simulink model "stg3"  (Simulink 7.0)
settings: Solver=ode45  StartTime=0.0  StopTime=100  RelTol=1e-3
libraries: xbsIndex_r4 x243, xps_library x11, casper_library x4
(part 1 of 2)
settings Model: Creator=dave  LastModifiedBy=dave

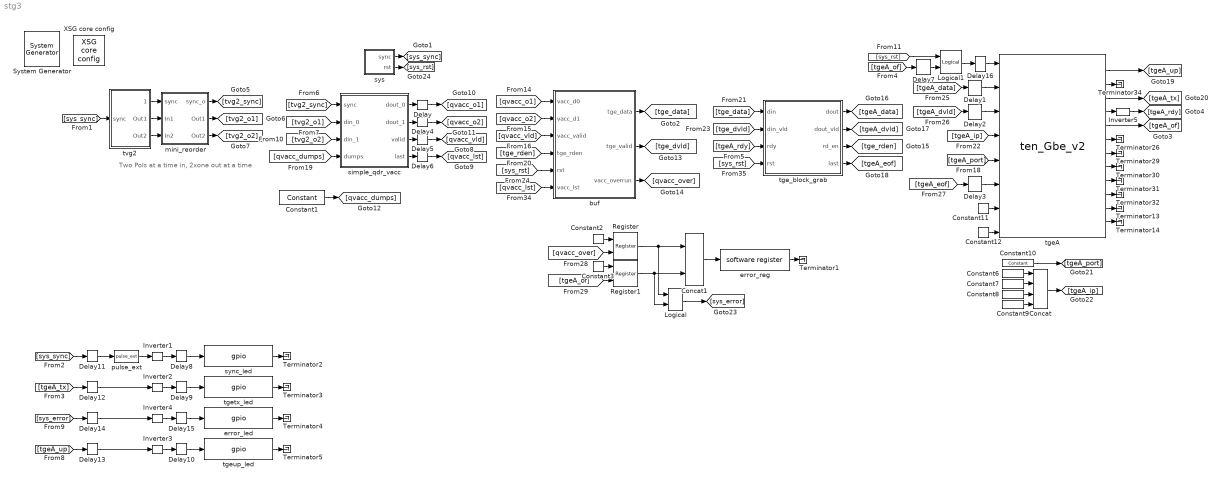
== system stg3 ==
  note: Two Pols at a time in,
      | 2xone out at a time
  " System Generator" : xbsIndex_r4/ System Generator  Tag=genX  SystemSampleTime=-1  xilinxfamily=virtex5  part=xc5vsx95t  speed=-1  package=ff1136  synthesis_tool=XST  clock_wrapper=Clock Enables  directory=./stg3/sysgen  testbench=off  simulink_period=1  sysclk_period=3.3333  dcm_input_clock_period=100  incr_netlist=off  trim_vbits=Everywhere in SubSystem  dbl_ovrd=According to Block Masks  core_generation=According to Block Masks  run_coregen=off  deprecated_control=off  eval_field=0  block_type=sysgen
      settings: block_version=10.1.3
  Concat : xbsIndex_r4/Concat  num_inputs=4  dbl_ovrd=off  block_type=concat
      settings: block_version=10.1.3
  Concat1 : xbsIndex_r4/Concat  num_inputs=2  dbl_ovrd=off  block_type=concat
      settings: block_version=10.1.3
  Constant1 : xbsIndex_r4/Constant  arith_type=Unsigned  const=(2^10)*(2^(10-1))*(2^9) - 2  n_bits=32  bin_pt=0  explicit_period=on  period=1  equ=P=C  opselect=C  inp2=PCIN>>17  opr=+  inp1=P  carry=CIN  dbl_ovrd=off  block_type=constant
  Constant10 : xbsIndex_r4/Constant  arith_type=Unsigned  const=10000  n_bits=16  bin_pt=0  explicit_period=off  period=1  equ=P=C  opselect=C  inp2=PCIN>>17  opr=+  inp1=P  carry=CIN  dbl_ovrd=off  block_type=constant
  Constant{2..3,11..12} (4 alike) : xbsIndex_r4/Constant  arith_type=Boolean  const=1  n_bits=16  bin_pt=14  explicit_period=off  period=1  equ=P=C  opselect=C  inp2=PCIN>>17  opr=+  inp1=P  carry=CIN  dbl_ovrd=off  block_type=constant
  Constant6 : xbsIndex_r4/Constant  arith_type=Unsigned  const=192  n_bits=8  bin_pt=0  explicit_period=off  period=1  equ=P=C  opselect=C  inp2=PCIN>>17  opr=+  inp1=P  carry=CIN  dbl_ovrd=off  block_type=constant
  Constant7 : xbsIndex_r4/Constant  arith_type=Unsigned  const=168  n_bits=8  bin_pt=0  explicit_period=off  period=1  equ=P=C  opselect=C  inp2=PCIN>>17  opr=+  inp1=P  carry=CIN  dbl_ovrd=off  block_type=constant
  Constant8 : xbsIndex_r4/Constant  arith_type=Unsigned  const=5  n_bits=8  bin_pt=0  explicit_period=off  period=1  equ=P=C  opselect=C  inp2=PCIN>>17  opr=+  inp1=P  carry=CIN  dbl_ovrd=off  block_type=constant
  Constant9 : xbsIndex_r4/Constant  arith_type=Unsigned  const=2  n_bits=8  bin_pt=0  explicit_period=off  period=1  equ=P=C  opselect=C  inp2=PCIN>>17  opr=+  inp1=P  carry=CIN  dbl_ovrd=off  block_type=constant
  Delay{,4..15} (13 alike) : xbsIndex_r4/Delay  en=off  latency=1  dbl_ovrd=off  reg_retiming=off  block_type=delay
  Delay{1..3,16} (4 alike) : xbsIndex_r4/Delay  en=off  latency=2  dbl_ovrd=off  reg_retiming=off  block_type=delay
  Inverter{1..5} (5 alike) : xbsIndex_r4/Inverter  en=off  latency=0  dbl_ovrd=off  block_type=inv
  Logical : xbsIndex_r4/Logical  logical_function=OR  inputs=2  en=off  latency=0  precision=Full  arith_type=Unsigned  n_bits=16  bin_pt=0  align_bp=on  dbl_ovrd=off  block_type=logical
  Logical1 : xbsIndex_r4/Logical  logical_function=OR  inputs=2  en=off  latency=0  precision=Full  arith_type=Unsigned  n_bits=16  bin_pt=0  align_bp=on  dbl_ovrd=off  block_type=logical
  Register : xbsIndex_r4/Register  init=0  rst=off  en=on  dbl_ovrd=off  block_type=register
  Register1 : xbsIndex_r4/Register  init=0  rst=off  en=on  dbl_ovrd=off  block_type=register
  Terminator{1..5,13..14,26,29..32,34} (13 alike) : Terminator
  XSG core config : xps_library/XSG core config  Tag=xps:xsg  SystemSampleTime=-1  hw_sys=ROACH:sx95t  ibob_linux=off  clk_src=arb_clk  iBOB_clk_src=sys_clk  BEE2_ctrl_clk_src=sys_clk  BEE2_usr_clk_src=sys_clk  ROACH_clk_src=arb_clk  CORR_clk_src=sys_clk  gpio_clk_io_group=iBOB:sma  gpio_clk_bit_index=0  clk_rate=300  sample_period=1  synthesis_tool=XST  mpc_type=powerpc440_ext
  buf : Subsystem  mask{fftsize=10, nochan=10}
      mask prompts: fftsize "fftsize (2^n)"; nochan "nochan (2^n)"
  error_led : xps_library/gpio  Tag=xps:gpio  SystemSampleTime=-1  io_group=ROACH:led  io_dir=out  arith_type=Boolean  bitwidth=1  bin_pt=0  bit_index=2  sample_period=1  use_single_ended=off  use_ddr=off  reg_iob=on  reg_clk_phase=0  termination=None
      link override convert: arith_type=Boolean  n_bits=1  bin_pt=0
  error_reg : xps_library/software register  Tag=xps:sw_reg  SystemSampleTime=-1  io_dir=To Processor  arith_type=Unsigned  bitwidth=32  bin_pt=0  sample_period=1  gw_name=stg3_error_reg_user_data_in
      link override convert: arith_type=Unsigned  n_bits=32  bin_pt=0
  mini_reorder : Subsystem
  pulse_ext : casper_library/Misc/pulse_ext  SystemSampleTime=-1  pulse_len=2^25
  simple_qdr_vacc : Subsystem  mask{n_chans=(2^10)*(2^(10-1)), which_qdr=1, add_lat=3}
      mask prompts: n_chans "Vector Length"; which_qdr "QDR Chip"; add_lat "add_latency"
      mask init:
      | set_param([gcb, '/qdr_delay'], 'which_qdr', sprintf('%d',which_qdr));
  sync_led : xps_library/gpio  Tag=xps:gpio  SystemSampleTime=-1  io_group=ROACH:led  io_dir=out  arith_type=Boolean  bitwidth=1  bin_pt=0  bit_index=0  sample_period=1  use_single_ended=off  use_ddr=off  reg_iob=on  reg_clk_phase=0  termination=None
      link override convert: arith_type=Boolean  n_bits=1  bin_pt=0
  sys : Subsystem
  tgeA : xps_library/ten_Gbe_v2  Tag=xps:tengbe_v2  SystemSampleTime=-1  port=0  rx_dist_ram=on  show_param=on  pre_emph=3  swing=800  fab_en=on  fab_mac=hex2dec('123456780000')  fab_ip=192*(2^24) + 168*(2^16) + 5*(2^8) + 20*(2^0)  fab_udp=10000  fab_gate=1  cpu_rx_en=off  cpu_tx_en=off
  tge_block_grab : Subsystem
  tgetx_led : xps_library/gpio  Tag=xps:gpio  SystemSampleTime=-1  io_group=ROACH:led  io_dir=out  arith_type=Boolean  bitwidth=1  bin_pt=0  bit_index=1  sample_period=1  use_single_ended=off  use_ddr=off  reg_iob=on  reg_clk_phase=0  termination=None
      link override convert: arith_type=Boolean  n_bits=1  bin_pt=0
  tgeup_led : xps_library/gpio  Tag=xps:gpio  SystemSampleTime=-1  io_group=ROACH:led  io_dir=out  arith_type=Boolean  bitwidth=1  bin_pt=0  bit_index=3  sample_period=1  use_single_ended=off  use_ddr=off  reg_iob=on  reg_clk_phase=0  termination=None
      link override convert: arith_type=Boolean  n_bits=1  bin_pt=0
  tvg2 : Subsystem  mask{fftsize=10, nochan=10, vaccwidth=18, dumps=9}
      mask prompts: fftsize "fftsize (2^n)"; nochan "nochan (2^n)"; dumps "dumps (2^n)"
  wires:
  [qvacc_dumps] -> simple_qdr_vacc/4(dumps)
  sys/1(sync) -> [sys_sync]
  [sys_sync] -> tvg2/1(sync)
  tgeA/1 -> [tgeA_up]
  tgeA/2 -> Terminator34/1
  tgeA/3 -> [tgeA_tx]
  [tgeA_ip] -> tgeA/4
  [tgeA_port] -> tgeA/5
  Constant6/1 -> Concat/1
  Constant7/1 -> Concat/2
  Constant8/1 -> Concat/3
  Constant9/1 -> Concat/4
  Concat/1 -> [tgeA_ip]
  Constant10/1 -> [tgeA_port]
  tgeA/4 -> Inverter5/1
  tgeA/6 -> Terminator26/1
  tgeA/7 -> Terminator29/1
  tgeA/8 -> Terminator30/1
  tgeA/9 -> Terminator31/1
  tgeA/10 -> Terminator32/1
  tgeA/11 -> Terminator13/1
  tgeA/12 -> Terminator14/1
  Constant11/1 -> tgeA/7
  Constant12/1 -> tgeA/8
  Delay1/1 -> tgeA/2
  Delay2/1 -> tgeA/3
  Delay3/1 -> tgeA/6
  tgeA/5 -> [tgeA_of]
  pulse_ext/1 -> Inverter1/1
  [sys_sync] -> Delay11/1
  [tgeA_tx] -> Delay12/1
  [tgeA_up] -> Delay13/1
  Delay8/1 -> sync_led/1
  Delay9/1 -> tgetx_led/1
  Delay10/1 -> tgeup_led/1
  Delay11/1 -> pulse_ext/1
  Delay12/1 -> Inverter2/1
  Delay13/1 -> Inverter3/1
  Inverter1/1 -> Delay8/1
  Inverter2/1 -> Delay9/1
  Inverter3/1 -> Delay10/1
  Delay15/1 -> error_led/1
  Inverter4/1 -> Delay15/1
  [sys_error] -> Delay14/1
  Delay14/1 -> Inverter4/1
  sync_led/1 -> Terminator2/1
  tgetx_led/1 -> Terminator3/1
  error_led/1 -> Terminator4/1
  tgeup_led/1 -> Terminator5/1
  [tgeA_of] -> Delay7/1
  Inverter5/1 -> [tgeA_rdy]
  [tgeA_rdy] -> tge_block_grab/3(rdy)
  [tvg2_sync] -> simple_qdr_vacc/1(sync)
  [tvg2_o1] -> simple_qdr_vacc/2(din_0)
  [tvg2_o2] -> simple_qdr_vacc/3(din_1)
  simple_qdr_vacc/1(dout_0) -> Delay/1
  simple_qdr_vacc/2(dout_1) -> Delay4/1
  simple_qdr_vacc/3(valid) -> Delay5/1
  Constant1/1 -> [qvacc_dumps]
  buf/1(tge_data) -> [tge_data]
  buf/2(tge_valid) -> [tge_dvld]
  buf/3(vacc_overrun) -> [qvacc_over]
  [tge_data] -> tge_block_grab/1(din)
  [tge_dvld] -> tge_block_grab/2(din_vld)
  tge_block_grab/3(rd_en) -> [tge_rden]
  tge_block_grab/1(dout) -> [tgeA_data]
  tge_block_grab/2(dout_vld) -> [tgeA_dvld]
  tge_block_grab/4(last) -> [tgeA_eof]
  [tgeA_data] -> Delay1/1
  [tgeA_dvld] -> Delay2/1
  [tgeA_eof] -> Delay3/1
  [qvacc_over] -> Register/2
  Constant2/1 -> Register/1
  [tgeA_of] -> Register1/2
  Constant3/1 -> Register1/1
  Register/1 -> Concat1/1, Logical/1
  Register1/1 -> Concat1/2, Logical/2
  Logical/1 -> [sys_error]
  error_reg/1 -> Terminator1/1
  Concat1/1 -> error_reg/1
  Delay/1 -> [qvacc_o1]
  Delay4/1 -> [qvacc_o2]
  tvg2/1(sync_o) -> mini_reorder/1(sync)
  tvg2/2(Out1) -> mini_reorder/2(In1)
  tvg2/3(Out2) -> mini_reorder/3(In2)
  mini_reorder/1(sync_o) -> [tvg2_sync]
  mini_reorder/2(Out1) -> [tvg2_o1]
  mini_reorder/3(Out2) -> [tvg2_o2]
  Delay5/1 -> [qvacc_vld]
  Delay6/1 -> [qvacc_lst]
  simple_qdr_vacc/4(last) -> Delay6/1
  sys/2(rst) -> [sys_rst]
  [qvacc_o1] -> buf/1(vacc_d0)
  [qvacc_o2] -> buf/2(vacc_d1)
  [qvacc_vld] -> buf/3(vacc_valid)
  [tge_rden] -> buf/4(tge_rden)
  [sys_rst] -> buf/5(rst)
  [qvacc_lst] -> buf/6(vacc_lst)
  [sys_rst] -> tge_block_grab/4(rst)
  [sys_rst] -> Logical1/1
  Delay7/1 -> Logical1/2
  Logical1/1 -> Delay16/1
  Delay16/1 -> tgeA/1

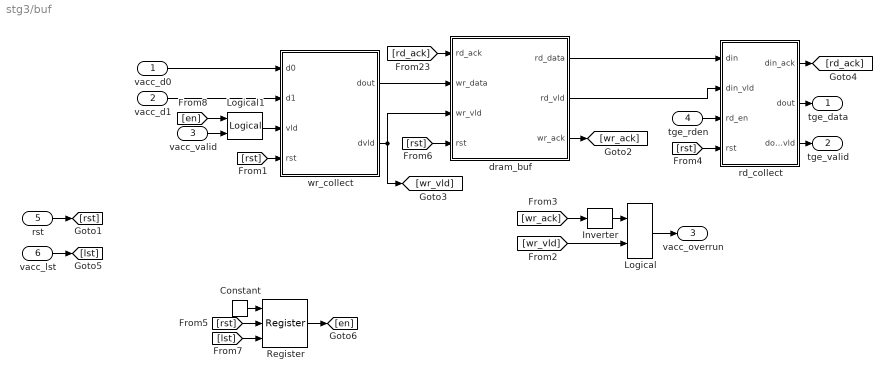
== system stg3/buf ==
  vacc_d0 : Inport
  vacc_d1 : Inport  Port=2
  vacc_valid : Inport  Port=3
  tge_rden : Inport  Port=4
  rst : Inport  Port=5
  vacc_lst : Inport  Port=6
  Constant : xbsIndex_r4/Constant  arith_type=Boolean  const=1  n_bits=16  bin_pt=14  explicit_period=off  period=1  equ=P=C  opselect=C  inp2=PCIN>>17  opr=+  inp1=P  carry=CIN  dbl_ovrd=off  block_type=constant
  Inverter : xbsIndex_r4/Inverter  en=off  latency=0  dbl_ovrd=off  block_type=inv
  Logical : xbsIndex_r4/Logical  logical_function=AND  inputs=2  en=off  latency=0  precision=Full  arith_type=Unsigned  n_bits=16  bin_pt=0  align_bp=on  dbl_ovrd=off  block_type=logical
  Logical1 : xbsIndex_r4/Logical  logical_function=AND  inputs=2  en=off  latency=0  precision=Full  arith_type=Unsigned  n_bits=16  bin_pt=0  align_bp=on  dbl_ovrd=off  block_type=logical
  Register : xbsIndex_r4/Register  init=0  rst=on  en=on  dbl_ovrd=off  block_type=register
  dram_buf : Subsystem  mask{block_size=fftsize+(nochan-1)-2}
      mask prompts: block_size "Block Size (2^n)"
  rd_collect : Subsystem
  wr_collect : Subsystem
  tge_data : Outport
  tge_valid : Outport  Port=2
  vacc_overrun : Outport  Port=3
  wires:
  vacc_d0/1 -> wr_collect/1(d0)
  vacc_d1/1 -> wr_collect/2(d1)
  rd_collect/2(dout) -> tge_data/1
  rd_collect/3(dout_vld) -> tge_valid/1
  wr_collect/1(dout) -> dram_buf/2(wr_data)
  wr_collect/2(dvld) -> dram_buf/3(wr_vld), [wr_vld]
  tge_rden/1 -> rd_collect/3(rd_en)
  Inverter/1 -> Logical/1
  Logical/1 -> vacc_overrun/1
  rd_collect/1(din_ack) -> [rd_ack]
  [rd_ack] -> dram_buf/1(rd_ack)
  dram_buf/3(wr_ack) -> [wr_ack]
  [wr_ack] -> Inverter/1
  [wr_vld] -> Logical/2
  dram_buf/1(rd_data) -> rd_collect/1(din)
  dram_buf/2(rd_vld) -> rd_collect/2(din_vld)
  rst/1 -> [rst]
  [rst] -> wr_collect/4(rst)
  [rst] -> dram_buf/4(rst)
  [rst] -> rd_collect/4(rst)
  vacc_lst/1 -> [lst]
  Constant/1 -> Register/1
  [rst] -> Register/2
  [lst] -> Register/3
  Register/1 -> [en]
  [en] -> Logical1/1
  Logical1/1 -> wr_collect/3(vld)
  vacc_valid/1 -> Logical1/2

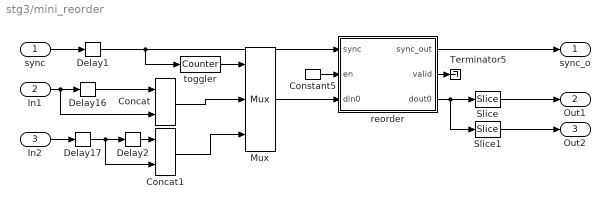
== system stg3/mini_reorder ==
  sync : Inport
  In1 : Inport  Port=2
  In2 : Inport  Port=3
  Concat : xbsIndex_r4/Concat  num_inputs=2  dbl_ovrd=off  block_type=concat
      settings: block_version=10.1.3
  Concat1 : xbsIndex_r4/Concat  num_inputs=2  dbl_ovrd=off  block_type=concat
      settings: block_version=10.1.3
  Constant5 : xbsIndex_r4/Constant  arith_type=Boolean  const=1  n_bits=1  bin_pt=0  explicit_period=on  period=1  equ=P=C  opselect=C  inp2=PCIN>>17  opr=+  inp1=P  carry=CIN  dbl_ovrd=off  block_type=constant
  Delay{1..2,16..17} (4 alike) : xbsIndex_r4/Delay  en=off  latency=1  dbl_ovrd=off  reg_retiming=off  block_type=delay
  Mux : xbsIndex_r4/Mux  inputs=2  en=off  latency=0  precision=Full  arith_type=Unsigned  n_bits=16  bin_pt=14  quantization=Truncate  overflow=Wrap  dbl_ovrd=off  block_type=mux
  Slice : xbsIndex_r4/Slice  nbits=18  boolean_output=off  mode=Lower Bit Location + Width  bit1=0  base1=LSB of Input  bit0=18  base0=LSB of Input  dbl_ovrd=off  block_type=slice
      settings: infoedit="Extracts a given range of bits from each input sample and presents it at the output.  The output type is ordinarily unsigned with binary point at zero, but can be Boolean when the slice is one bit wide.<P><P>Hardware notes: In hardware this block costs nothing."  block_version=10.1.3
  Slice1 : xbsIndex_r4/Slice  nbits=18  boolean_output=off  mode=Lower Bit Location + Width  bit1=0  base1=LSB of Input  bit0=0  base0=LSB of Input  dbl_ovrd=off  block_type=slice
      settings: infoedit="Extracts a given range of bits from each input sample and presents it at the output.  The output type is ordinarily unsigned with binary point at zero, but can be Boolean when the slice is one bit wide.<P><P>Hardware notes: In hardware this block costs nothing."  block_version=10.1.3
  Terminator5 : Terminator
  reorder : Subsystem  AncestorBlock=casper_library/Reorder/reorder  mask(reorder){map=getfield( getfield( get_param( gcb,'UserData' ), 'parameters'),'map'), n_inputs=1, bram_latency=3, map_latency=3, double_buffer=0}
      mask prompts: map "Output Order:"; n_inputs "Number of inputs"; bram_latency "BRAM Latency"; map_latency "Map Latency"; double_buffer "Double Buffer"
      mask init:
      | reorder_init(gcb, ...
      |     'map', map, ...
      |     'n_inputs', n_inputs, ...
      |     'bram_latency', bram_latency, ...
      |     'map_latency', map_latency, ...
      |     'double_buffer', double_buffer);
      settings: AttributesFormatString=order=10
      mask Help: eval('xlWeb([getenv(''MLIB_ROOT''), ''\doc\htmlblocks\sp_reorder\sp_reorder.html''])')
  toggler : xbsIndex_r4/Counter  cnt_type=Free Running  cnt_to=Inf  operation=Up  start_count=0  cnt_by_val=1  arith_type=Unsigned  n_bits=1  bin_pt=0  load_pin=off  rst=on  en=off  explicit_period=on  period=1  dbl_ovrd=off  use_behavioral_HDL=off  use_rpm=off  implementation=Fabric  block_type=counter
  sync_o : Outport
  Out1 : Outport  Port=2
  Out2 : Outport  Port=3
  wires:
  toggler/1 -> Mux/1
  sync/1 -> Delay1/1
  In1/1 -> Delay16/1, Concat/2
  In2/1 -> Delay17/1
  Delay1/1 -> toggler/1, reorder/1(sync)
  Delay16/1 -> Concat/1
  Delay17/1 -> Delay2/1, Concat1/2
  Delay2/1 -> Concat1/1
  Concat1/1 -> Mux/3
  Concat/1 -> Mux/2
  Slice/1 -> Out1/1
  Slice1/1 -> Out2/1
  Constant5/1 -> reorder/2(en)
  Mux/1 -> reorder/3(din0)
  reorder/1(sync_out) -> sync_o/1
  reorder/2(valid) -> Terminator5/1
  reorder/3(dout0) -> Slice/1, Slice1/1

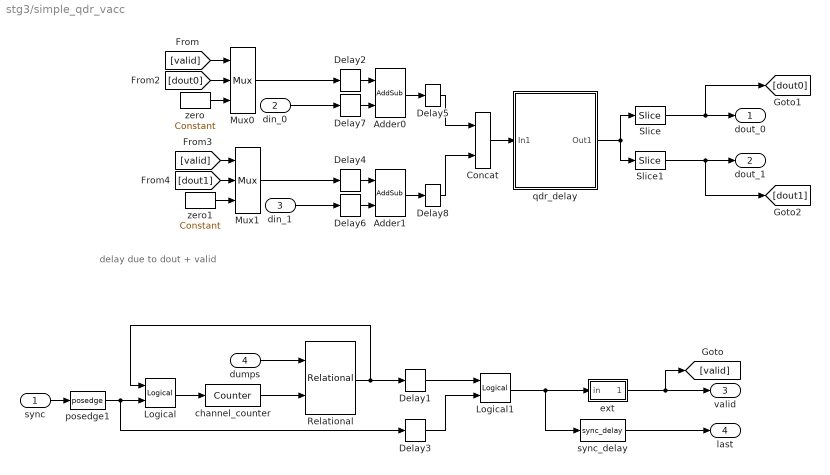
== system stg3/simple_qdr_vacc ==
  note: delay due to
      | dout + valid
  sync : Inport
  din_0 : Inport  Port=2
  din_1 : Inport  Port=3
  dumps : Inport  Port=4
  Adder0 : xbsIndex_r4/AddSub  mode=Addition  use_carryin=off  use_carryout=off  en=off  latency=add_lat-1  precision=User Defined  arith_type=Unsigned  n_bits=18  bin_pt=0  quantization=Truncate  overflow=Saturate  dbl_ovrd=off  use_behavioral_HDL=on  pipelined=off  use_rpm=on  hw_selection=Fabric  block_type=addsub
      settings: xl_area=[0, 0, 0, 0, 0, 0, 0]  block_version=10.1.3
  Adder1 : xbsIndex_r4/AddSub  mode=Addition  use_carryin=off  use_carryout=off  en=off  latency=add_lat-1  precision=User Defined  arith_type=Unsigned  n_bits=18  bin_pt=0  quantization=Truncate  overflow=Saturate  dbl_ovrd=off  use_behavioral_HDL=on  pipelined=off  use_rpm=on  hw_selection=Fabric  block_type=addsub
      settings: xl_area=[0, 0, 0, 0, 0, 0, 0]  block_version=10.1.3
  Concat : xbsIndex_r4/Concat  num_inputs=2  dbl_ovrd=off  block_type=concat
      settings: block_version=10.1.3
  Delay{1..4,6..7} (6 alike) : xbsIndex_r4/Delay  en=off  latency=1  dbl_ovrd=off  reg_retiming=off  block_type=delay
  Delay5 : xbsIndex_r4/Delay  en=off  latency=add_lat>1  dbl_ovrd=off  reg_retiming=off  block_type=delay
  Delay8 : xbsIndex_r4/Delay  en=off  latency=add_lat>1  dbl_ovrd=off  reg_retiming=off  block_type=delay
  Logical : xbsIndex_r4/Logical  logical_function=OR  inputs=2  en=off  latency=0  precision=Full  arith_type=Unsigned  n_bits=16  bin_pt=0  align_bp=on  dbl_ovrd=off  block_type=logical
  Logical1 : xbsIndex_r4/Logical  logical_function=OR  inputs=2  en=off  latency=0  precision=Full  arith_type=Unsigned  n_bits=16  bin_pt=0  align_bp=on  dbl_ovrd=off  block_type=logical
  Mux0 : xbsIndex_r4/Mux  inputs=2  en=off  latency=0  precision=Full  arith_type="Signed  (2's comp)"  n_bits=8  bin_pt=2  quantization=Truncate  overflow=Wrap  dbl_ovrd=off  block_type=mux
      settings: xl_area=[0, 0, 0, 0, 0, 0, 0]
  Mux1 : xbsIndex_r4/Mux  inputs=2  en=off  latency=0  precision=Full  arith_type="Signed  (2's comp)"  n_bits=8  bin_pt=2  quantization=Truncate  overflow=Wrap  dbl_ovrd=off  block_type=mux
      settings: xl_area=[0, 0, 0, 0, 0, 0, 0]
  Relational : xbsIndex_r4/Relational  mode=a=b  en=off  latency=1  dbl_ovrd=off  block_type=relational
      settings: block_version=10.1.3
  Slice : xbsIndex_r4/Slice  nbits=18  boolean_output=off  mode=Lower Bit Location + Width  bit1=0  base1=MSB of Input  bit0=18  base0=LSB of Input  dbl_ovrd=off  block_type=slice
      settings: infoedit="Extracts a given range of bits from each input sample and presents it at the output.  The output type is ordinarily unsigned with binary point at zero, but can be Boolean when the slice is one bit wide.<P><P>Hardware notes: In hardware this block costs nothing."  block_version=10.1.3
  Slice1 : xbsIndex_r4/Slice  nbits=18  boolean_output=off  mode=Lower Bit Location + Width  bit1=0  base1=MSB of Input  bit0=0  base0=LSB of Input  dbl_ovrd=off  block_type=slice
      settings: infoedit="Extracts a given range of bits from each input sample and presents it at the output.  The output type is ordinarily unsigned with binary point at zero, but can be Boolean when the slice is one bit wide.<P><P>Hardware notes: In hardware this block costs nothing."  block_version=10.1.3
  channel_counter : xbsIndex_r4/Counter  cnt_type=Free Running  cnt_to=Inf  operation=Up  start_count=0  cnt_by_val=1  arith_type=Unsigned  n_bits=32  bin_pt=0  load_pin=off  rst=on  en=off  explicit_period=on  period=1  dbl_ovrd=off  use_behavioral_HDL=off  use_rpm=off  implementation=Fabric  block_type=counter
  ext : Subsystem  mask(pulse_ext){pulse_len=n_chans}
      mask prompts: pulse_len "Length of Pulse"
      mask help:
      | Extends a boolean signal to be high for the specified number of clocks after
      | the last high input.
      mask init:
      | bits = ceil(log2(pulse_len))+1;
      mask Help: eval('xlWeb([getenv(''MLIB_ROOT''), ''\doc\htmlblocks\sp_pulse_ext\sp_pulse_ext.html''])')
  posedge1 : casper_library/Misc/posedge  Tag=Rising Edge Detector  SystemSampleTime=-1
  qdr_delay : Subsystem  mask{which_qdr=1, delay=n_chans - add_lat - 1}
      mask prompts: which_qdr "QDR Chip"
      mask init:
      | bits = ceil(log2(max(2,(ceil((max(0,delay-10)/2)*2)))));
      | set_param([gcb, '/qdr'], 'which_qdr', sprintf('qdr%d',which_qdr));
  sync_delay : casper_library/Delays/sync_delay  SystemSampleTime=-1  DelayLen=n_chans-1
  zero : xbsIndex_r4/Constant  arith_type=Unsigned  const=0  n_bits=18  bin_pt=0  explicit_period=on  period=1  equ=P=C  opselect=C  inp2=PCIN>>17  opr=+  inp1=P  carry=CIN  dbl_ovrd=off  block_type=constant
  zero1 : xbsIndex_r4/Constant  arith_type=Unsigned  const=0  n_bits=18  bin_pt=0  explicit_period=on  period=1  equ=P=C  opselect=C  inp2=PCIN>>17  opr=+  inp1=P  carry=CIN  dbl_ovrd=off  block_type=constant
  dout_0 : Outport
  dout_1 : Outport  Port=2
  valid : Outport  Port=3
  last : Outport  Port=4
  wires:
  Logical1/1 -> sync_delay/1, ext/1(in)
  Delay3/1 -> Logical1/2
  Delay1/1 -> Logical1/1
  Delay6/1 -> Adder1/2
  Delay4/1 -> Adder1/1
  Delay7/1 -> Adder0/2
  Delay2/1 -> Adder0/1
  Adder1/1 -> Delay8/1
  Adder0/1 -> Delay5/1
  dumps/1 -> Relational/1
  sync_delay/1 -> last/1
  [dout1] -> Mux1/2
  [valid] -> Mux1/1
  [dout0] -> Mux0/2
  [valid] -> Mux0/1
  zero1/1 -> Mux1/3
  ext/1(out) -> [valid], valid/1
  Mux0/1 -> Delay2/1
  Slice1/1 -> [dout1], dout_1/1
  Slice/1 -> [dout0], dout_0/1
  posedge1/1 -> Delay3/1, Logical/2
  Relational/1 -> Delay1/1, Logical/1
  Logical/1 -> channel_counter/1
  channel_counter/1 -> Relational/2
  sync/1 -> posedge1/1
  qdr_delay/1(Out1) -> Slice/1, Slice1/1
  Concat/1 -> qdr_delay/1(In1)
  din_1/1 -> Delay6/1
  din_0/1 -> Delay7/1
  Mux1/1 -> Delay4/1
  zero/1 -> Mux0/3
  Delay5/1 -> Concat/1
  Delay8/1 -> Concat/2

== system stg3/sys ==
  Constant1 : xbsIndex_r4/Constant  arith_type=Unsigned  const=2^5-1  n_bits=5  bin_pt=0  explicit_period=on  period=1  equ=P=C  opselect=C  inp2=PCIN>>17  opr=+  inp1=P  carry=CIN  dbl_ovrd=off  block_type=constant
  Constant4 : Constant  Value=0  OutDataType=sfix(16)  OutScaling=2^0
  Constant5 : xbsIndex_r4/Constant  arith_type=Unsigned  const=2^5-2  n_bits=5  bin_pt=0  explicit_period=on  period=1  equ=P=C  opselect=C  inp2=PCIN>>17  opr=+  inp1=P  carry=CIN  dbl_ovrd=off  block_type=constant
  Delay18 : xbsIndex_r4/Delay  en=off  latency=1  dbl_ovrd=off  reg_retiming=off  block_type=delay
  Delay19 : xbsIndex_r4/Delay  en=off  latency=1  dbl_ovrd=off  reg_retiming=off  block_type=delay
  Relational : xbsIndex_r4/Relational  mode=a=b  en=off  latency=0  dbl_ovrd=off  block_type=relational
      settings: block_version=10.1.3
  Relational1 : xbsIndex_r4/Relational  mode=a!=b  en=off  latency=0  dbl_ovrd=off  block_type=relational
      settings: block_version=10.1.3
  Slice : xbsIndex_r4/Slice  nbits=1  boolean_output=on  mode=Lower Bit Location + Width  bit1=0  base1=MSB of Input  bit0=0  base0=LSB of Input  dbl_ovrd=off  block_type=slice
      settings: infoedit="Extracts a given range of bits from each input sample and presents it at the output.  The output type is ordinarily unsigned with binary point at zero, but can be Boolean when the slice is one bit wide.<P><P>Hardware notes: In hardware this block costs nothing."  block_version=10.1.3
  reset_reg : xps_library/software register  Tag=xps:sw_reg  SystemSampleTime=-1  io_dir=From Processor  arith_type=Unsigned  bitwidth=32  bin_pt=0  sample_period=1  gw_name=stg3_sys_reset_reg_user_data_out
      link override qdr_vacc_dram_buf_tv_Subsystem_reset_reg_user_data_out: arith_type=Unsigned  n_bits=32  bin_pt=0  period=1
      link override qdr_vacc_dram_buf_tv_reset_reg_user_data_out: arith_type=Unsigned  n_bits=32  bin_pt=0  period=1
      link override qdr_vacc_dram_buf_tv_sys_reset_reg_user_data_out: arith_type=Unsigned  n_bits=32  bin_pt=0  period=1
      link override qdr_vacc_dram_buf_tv_tvg2_chan_user_data_out: arith_type=Unsigned  n_bits=32  bin_pt=0  period=1
      link override stg3_backup_sys_reset_reg_user_data_out: arith_type=Unsigned  n_bits=32  bin_pt=0  period=1
      link override stg3_sys_reset_reg_user_data_out: arith_type=Unsigned  n_bits=32  bin_pt=0  period=1
  sync_counter : xbsIndex_r4/Counter  cnt_type=Free Running  cnt_to=15  operation=Up  start_count=0  cnt_by_val=1  arith_type=Unsigned  n_bits=5  bin_pt=0  load_pin=off  rst=on  en=on  explicit_period=on  period=1  dbl_ovrd=off  use_behavioral_HDL=off  use_rpm=off  implementation=Fabric  block_type=counter
  sync : Outport
  rst : Outport  Port=2
  wires:
  sync_counter/1 -> Relational/1, Relational1/1
  Constant5/1 -> Relational/2
  Constant4/1 -> reset_reg/1
  reset_reg/1 -> Slice/1
  Relational/1 -> Delay19/1
  Slice/1 -> sync_counter/1, Delay18/1
  Constant1/1 -> Relational1/2
  Relational1/1 -> sync_counter/2
  Delay18/1 -> rst/1
  Delay19/1 -> sync/1

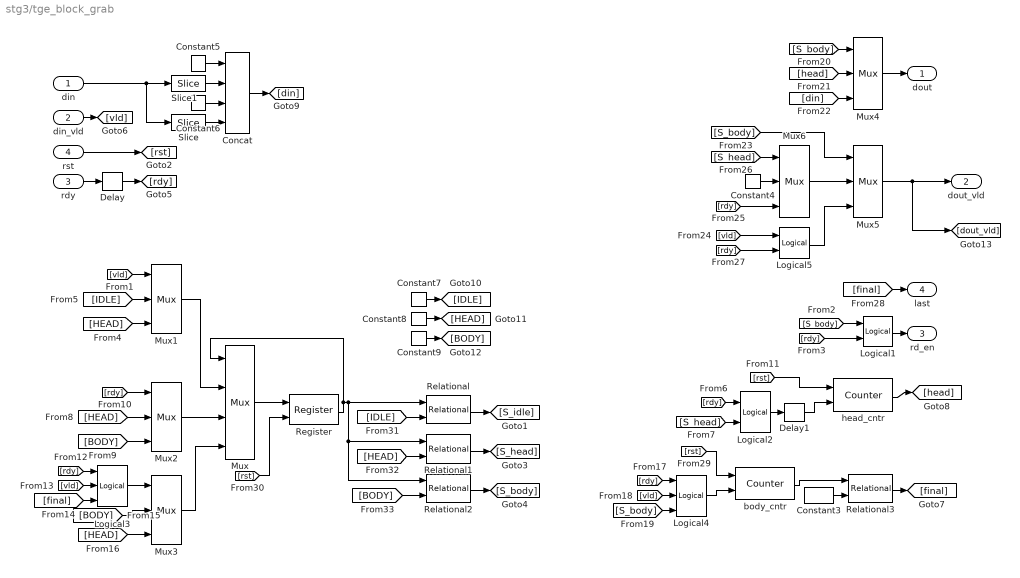
== system stg3/tge_block_grab ==
  din : Inport
  din_vld : Inport  Port=2
  rdy : Inport  Port=3
  rst : Inport  Port=4
  Concat : xbsIndex_r4/Concat  num_inputs=4  dbl_ovrd=off  block_type=concat
      settings: block_version=10.1.3
  Constant3 : xbsIndex_r4/Constant  arith_type=Unsigned  const=2^9-1  n_bits=9  bin_pt=0  explicit_period=off  period=1  equ=P=C  opselect=C  inp2=PCIN>>17  opr=+  inp1=P  carry=CIN  dbl_ovrd=off  block_type=constant
  Constant4 : xbsIndex_r4/Constant  arith_type=Boolean  const=0  n_bits=2  bin_pt=0  explicit_period=off  period=1  equ=P=C  opselect=C  inp2=PCIN>>17  opr=+  inp1=P  carry=CIN  dbl_ovrd=off  block_type=constant
  Constant5 : xbsIndex_r4/Constant  arith_type=Unsigned  const=0  n_bits=14  bin_pt=0  explicit_period=off  period=1  equ=P=C  opselect=C  inp2=PCIN>>17  opr=+  inp1=P  carry=CIN  dbl_ovrd=off  block_type=constant
  Constant6 : xbsIndex_r4/Constant  arith_type=Unsigned  const=0  n_bits=14  bin_pt=0  explicit_period=off  period=1  equ=P=C  opselect=C  inp2=PCIN>>17  opr=+  inp1=P  carry=CIN  dbl_ovrd=off  block_type=constant
  Constant7 : xbsIndex_r4/Constant  arith_type=Unsigned  const=0  n_bits=2  bin_pt=0  explicit_period=off  period=1  equ=P=C  opselect=C  inp2=PCIN>>17  opr=+  inp1=P  carry=CIN  dbl_ovrd=off  block_type=constant
  Constant8 : xbsIndex_r4/Constant  arith_type=Unsigned  const=1  n_bits=2  bin_pt=0  explicit_period=off  period=1  equ=P=C  opselect=C  inp2=PCIN>>17  opr=+  inp1=P  carry=CIN  dbl_ovrd=off  block_type=constant
  Constant9 : xbsIndex_r4/Constant  arith_type=Unsigned  const=2  n_bits=2  bin_pt=0  explicit_period=off  period=1  equ=P=C  opselect=C  inp2=PCIN>>17  opr=+  inp1=P  carry=CIN  dbl_ovrd=off  block_type=constant
  Delay : xbsIndex_r4/Delay  en=off  latency=1  dbl_ovrd=off  reg_retiming=off  block_type=delay
  Delay1 : xbsIndex_r4/Delay  en=off  latency=1  dbl_ovrd=off  reg_retiming=off  block_type=delay
  Logical1 : xbsIndex_r4/Logical  logical_function=AND  inputs=2  en=off  latency=0  precision=Full  arith_type=Unsigned  n_bits=16  bin_pt=0  align_bp=on  dbl_ovrd=off  block_type=logical
  Logical2 : xbsIndex_r4/Logical  logical_function=AND  inputs=2  en=off  latency=0  precision=Full  arith_type=Unsigned  n_bits=16  bin_pt=0  align_bp=on  dbl_ovrd=off  block_type=logical
  Logical3 : xbsIndex_r4/Logical  logical_function=AND  inputs=3  en=off  latency=0  precision=Full  arith_type=Unsigned  n_bits=16  bin_pt=0  align_bp=on  dbl_ovrd=off  block_type=logical
  Logical4 : xbsIndex_r4/Logical  logical_function=AND  inputs=3  en=off  latency=0  precision=Full  arith_type=Unsigned  n_bits=16  bin_pt=0  align_bp=on  dbl_ovrd=off  block_type=logical
  Logical5 : xbsIndex_r4/Logical  logical_function=AND  inputs=2  en=off  latency=0  precision=Full  arith_type=Unsigned  n_bits=16  bin_pt=0  align_bp=on  dbl_ovrd=off  block_type=logical
  Mux : xbsIndex_r4/Mux  inputs=3  en=off  latency=0  precision=Full  arith_type=Unsigned  n_bits=16  bin_pt=14  quantization=Truncate  overflow=Wrap  dbl_ovrd=off  block_type=mux
  Mux{1..6} (6 alike) : xbsIndex_r4/Mux  inputs=2  en=off  latency=0  precision=Full  arith_type=Unsigned  n_bits=16  bin_pt=14  quantization=Truncate  overflow=Wrap  dbl_ovrd=off  block_type=mux
  Register : xbsIndex_r4/Register  init=0  rst=on  en=off  dbl_ovrd=off  block_type=register
  Relational{,1..3} (4 alike) : xbsIndex_r4/Relational  mode=a=b  en=off  latency=0  dbl_ovrd=off  block_type=relational
      settings: block_version=10.1.3
  Slice : xbsIndex_r4/Slice  nbits=18  boolean_output=off  mode=Lower Bit Location + Width  bit1=0  base1=LSB of Input  bit0=0  base0=LSB of Input  dbl_ovrd=off  block_type=slice
      settings: infoedit="Extracts a given range of bits from each input sample and presents it at the output.  The output type is ordinarily unsigned with binary point at zero, but can be Boolean when the slice is one bit wide.<P><P>Hardware notes: In hardware this block costs nothing."  block_version=10.1.3
  Slice1 : xbsIndex_r4/Slice  nbits=18  boolean_output=off  mode=Lower Bit Location + Width  bit1=0  base1=LSB of Input  bit0=18  base0=LSB of Input  dbl_ovrd=off  block_type=slice
      settings: infoedit="Extracts a given range of bits from each input sample and presents it at the output.  The output type is ordinarily unsigned with binary point at zero, but can be Boolean when the slice is one bit wide.<P><P>Hardware notes: In hardware this block costs nothing."  block_version=10.1.3
  body_cntr : xbsIndex_r4/Counter  cnt_type=Free Running  cnt_to=Inf  operation=Up  start_count=0  cnt_by_val=1  arith_type=Unsigned  n_bits=9  bin_pt=0  load_pin=off  rst=on  en=on  explicit_period=on  period=1  dbl_ovrd=off  use_behavioral_HDL=off  use_rpm=off  implementation=Fabric  block_type=counter
  head_cntr : xbsIndex_r4/Counter  cnt_type=Free Running  cnt_to=Inf  operation=Up  start_count=0  cnt_by_val=1  arith_type=Unsigned  n_bits=64  bin_pt=0  load_pin=off  rst=on  en=on  explicit_period=on  period=1  dbl_ovrd=off  use_behavioral_HDL=off  use_rpm=off  implementation=Fabric  block_type=counter
  dout : Outport
  dout_vld : Outport  Port=2
  rd_en : Outport  Port=3
  last : Outport  Port=4
  wires:
  Register/1 -> Relational2/1, Relational1/1, Relational/1, Mux/1
  Relational/1 -> [S_idle]
  Relational1/1 -> [S_head]
  Relational2/1 -> [S_body]
  rdy/1 -> Delay/1
  [rdy] -> Logical1/2
  Logical1/1 -> rd_en/1
  Logical2/1 -> Delay1/1
  Delay/1 -> [rdy]
  [S_body] -> Logical1/1
  [rdy] -> Logical2/1
  [S_head] -> Logical2/2
  Mux/1 -> Register/1
  din_vld/1 -> [vld]
  [vld] -> Mux1/1
  [HEAD] -> Mux1/3
  [IDLE] -> Mux1/2
  Mux1/1 -> Mux/2
  Mux2/1 -> Mux/3
  [HEAD] -> Mux2/2
  [BODY] -> Mux2/3
  [rdy] -> Mux2/1
  [rdy] -> Logical3/1
  [vld] -> Logical3/2
  [final] -> Logical3/3
  Logical3/1 -> Mux3/1
  [BODY] -> Mux3/2
  [HEAD] -> Mux3/3
  head_cntr/1 -> [head]
  Constant3/1 -> Relational3/2
  body_cntr/1 -> Relational3/1
  [rdy] -> Logical4/1
  [vld] -> Logical4/2
  [S_body] -> Logical4/3
  Relational3/1 -> [final]
  Mux3/1 -> Mux/4
  [S_body] -> Mux4/1
  [head] -> Mux4/2
  [din] -> Mux4/3
  Mux4/1 -> dout/1
  [S_body] -> Mux5/1
  Mux5/1 -> dout_vld/1, [dout_vld]
  Mux6/1 -> Mux5/2
  [S_head] -> Mux6/1
  Constant4/1 -> Mux6/2
  [rdy] -> Logical5/2
  [vld] -> Logical5/1
  Logical5/1 -> Mux5/3
  [rdy] -> Mux6/3
  [final] -> last/1
  Concat/1 -> [din]
  Slice1/1 -> Concat/2
  Constant5/1 -> Concat/1
  Constant6/1 -> Concat/3
  din/1 -> Slice1/1, Slice/1
  Slice/1 -> Concat/4
  Constant7/1 -> [IDLE]
  Constant8/1 -> [HEAD]
  Constant9/1 -> [BODY]
  [IDLE] -> Relational/2
  [HEAD] -> Relational1/2
  [BODY] -> Relational2/2
  rst/1 -> [rst]
  [rst] -> head_cntr/1
  Delay1/1 -> head_cntr/2
  [rst] -> body_cntr/1
  Logical4/1 -> body_cntr/2
  [rst] -> Register/2

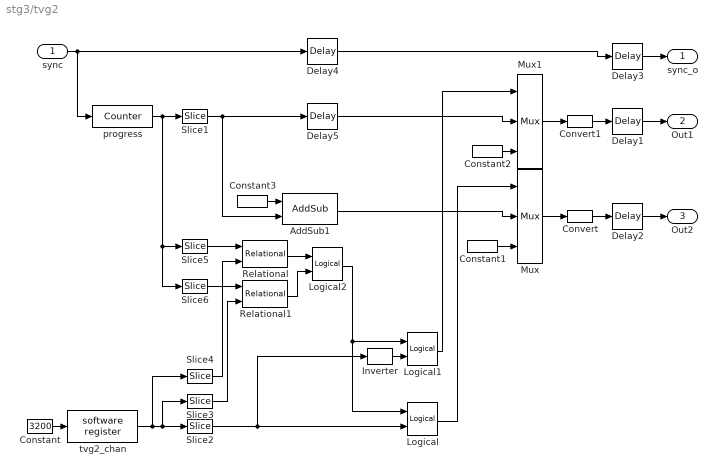
== system stg3/tvg2 ==
  sync : Inport  OutDataType=sfix(16)  OutScaling=2^0
  AddSub1 : xbsIndex_r4/AddSub  mode=Subtraction  use_carryin=off  use_carryout=off  en=off  latency=2  precision=Full  arith_type=Unsigned  n_bits=16  bin_pt=14  quantization=Truncate  overflow=Wrap  dbl_ovrd=off  use_behavioral_HDL=off  pipelined=off  use_rpm=on  hw_selection=Fabric  block_type=addsub
      settings: block_version=10.1.3
  Constant : Constant  Value=3200  OutDataType=sfix(16)  OutScaling=2^0
  Constant1 : xbsIndex_r4/Constant  arith_type=Unsigned  const=128  n_bits=7  bin_pt=0  explicit_period=on  period=1  equ=P=C  opselect=C  inp2=PCIN>>17  opr=+  inp1=P  carry=CIN  dbl_ovrd=off  block_type=constant
  Constant2 : xbsIndex_r4/Constant  arith_type=Unsigned  const=128  n_bits=7  bin_pt=0  explicit_period=on  period=1  equ=P=C  opselect=C  inp2=PCIN>>17  opr=+  inp1=P  carry=CIN  dbl_ovrd=off  block_type=constant
  Constant3 : xbsIndex_r4/Constant  arith_type=Unsigned  const=63  n_bits=6  bin_pt=0  explicit_period=on  period=1  equ=P=C  opselect=C  inp2=PCIN>>17  opr=+  inp1=P  carry=CIN  dbl_ovrd=off  block_type=constant
  Convert : xbsIndex_r4/Convert  arith_type=Unsigned  n_bits=vaccwidth  bin_pt=0  quantization=Truncate  overflow=Wrap  latency=0  dbl_ovrd=off  pipeline=off  block_type=convert
      settings: block_version=10.1.3
  Convert1 : xbsIndex_r4/Convert  arith_type=Unsigned  n_bits=vaccwidth  bin_pt=0  quantization=Truncate  overflow=Wrap  latency=0  dbl_ovrd=off  pipeline=off  block_type=convert
      settings: block_version=10.1.3
  Delay1 : xbsIndex_r4/Delay  en=off  latency=1  dbl_ovrd=off  reg_retiming=off  block_type=delay
  Delay2 : xbsIndex_r4/Delay  en=off  latency=1  dbl_ovrd=off  reg_retiming=off  block_type=delay
  Delay3 : xbsIndex_r4/Delay  en=off  latency=1  dbl_ovrd=off  reg_retiming=off  block_type=delay
  Delay4 : xbsIndex_r4/Delay  en=off  latency=2  dbl_ovrd=off  reg_retiming=off  block_type=delay
  Delay5 : xbsIndex_r4/Delay  en=off  latency=2  dbl_ovrd=off  reg_retiming=off  block_type=delay
  Inverter : xbsIndex_r4/Inverter  en=off  latency=0  dbl_ovrd=off  block_type=inv
  Logical : xbsIndex_r4/Logical  logical_function=AND  inputs=2  en=off  latency=1  precision=Full  arith_type=Unsigned  n_bits=16  bin_pt=0  align_bp=on  dbl_ovrd=off  block_type=logical
  Logical1 : xbsIndex_r4/Logical  logical_function=AND  inputs=2  en=off  latency=1  precision=Full  arith_type=Unsigned  n_bits=16  bin_pt=0  align_bp=on  dbl_ovrd=off  block_type=logical
  Logical2 : xbsIndex_r4/Logical  logical_function=AND  inputs=2  en=off  latency=0  precision=Full  arith_type=Unsigned  n_bits=16  bin_pt=0  align_bp=on  dbl_ovrd=off  block_type=logical
  Mux : xbsIndex_r4/Mux  inputs=2  en=off  latency=0  precision=Full  arith_type=Unsigned  n_bits=16  bin_pt=14  quantization=Truncate  overflow=Wrap  dbl_ovrd=off  block_type=mux
  Mux1 : xbsIndex_r4/Mux  inputs=2  en=off  latency=0  precision=Full  arith_type=Unsigned  n_bits=16  bin_pt=14  quantization=Truncate  overflow=Wrap  dbl_ovrd=off  block_type=mux
  Relational : xbsIndex_r4/Relational  mode=a=b  en=off  latency=1  dbl_ovrd=off  block_type=relational
      settings: block_version=10.1.3
  Relational1 : xbsIndex_r4/Relational  mode=a=b  en=off  latency=1  dbl_ovrd=off  block_type=relational
      settings: block_version=10.1.3
  Slice1 : xbsIndex_r4/Slice  nbits=fftsize-4  boolean_output=off  mode=Lower Bit Location + Width  bit1=0  base1=LSB of Input  bit0=4  base0=LSB of Input  dbl_ovrd=off  block_type=slice
      settings: infoedit="Extracts a given range of bits from each input sample and presents it at the output.  The output type is ordinarily unsigned with binary point at zero, but can be Boolean when the slice is one bit wide.<P><P>Hardware notes: In hardware this block costs nothing."  block_version=10.1.3
  Slice2 : xbsIndex_r4/Slice  nbits=1  boolean_output=on  mode=Lower Bit Location + Width  bit1=0  base1=LSB of Input  bit0=10  base0=LSB of Input  dbl_ovrd=off  block_type=slice
      settings: infoedit="Extracts a given range of bits from each input sample and presents it at the output.  The output type is ordinarily unsigned with binary point at zero, but can be Boolean when the slice is one bit wide.<P><P>Hardware notes: In hardware this block costs nothing."  block_version=10.1.3
  Slice3 : xbsIndex_r4/Slice  nbits=10-1  boolean_output=off  mode=Lower Bit Location + Width  bit1=0  base1=LSB of Input  bit0=11  base0=LSB of Input  dbl_ovrd=off  block_type=slice
      settings: infoedit="Extracts a given range of bits from each input sample and presents it at the output.  The output type is ordinarily unsigned with binary point at zero, but can be Boolean when the slice is one bit wide.<P><P>Hardware notes: In hardware this block costs nothing."  block_version=10.1.3
  Slice4 : xbsIndex_r4/Slice  nbits=fftsize  boolean_output=off  mode=Lower Bit Location + Width  bit1=0  base1=LSB of Input  bit0=0  base0=LSB of Input  dbl_ovrd=off  block_type=slice
      settings: infoedit="Extracts a given range of bits from each input sample and presents it at the output.  The output type is ordinarily unsigned with binary point at zero, but can be Boolean when the slice is one bit wide.<P><P>Hardware notes: In hardware this block costs nothing."  block_version=10.1.3
  Slice5 : xbsIndex_r4/Slice  nbits=fftsize  boolean_output=off  mode=Lower Bit Location + Width  bit1=0  base1=LSB of Input  bit0=0  base0=LSB of Input  dbl_ovrd=off  block_type=slice
      settings: infoedit="Extracts a given range of bits from each input sample and presents it at the output.  The output type is ordinarily unsigned with binary point at zero, but can be Boolean when the slice is one bit wide.<P><P>Hardware notes: In hardware this block costs nothing."  block_version=10.1.3
  Slice6 : xbsIndex_r4/Slice  nbits=nochan-1  boolean_output=off  mode=Lower Bit Location + Width  bit1=0  base1=LSB of Input  bit0=fftsize  base0=LSB of Input  dbl_ovrd=off  block_type=slice
      settings: infoedit="Extracts a given range of bits from each input sample and presents it at the output.  The output type is ordinarily unsigned with binary point at zero, but can be Boolean when the slice is one bit wide.<P><P>Hardware notes: In hardware this block costs nothing."  block_version=10.1.3
  progress : xbsIndex_r4/Counter  cnt_type=Free Running  cnt_to=Inf  operation=Up  start_count=0  cnt_by_val=1  arith_type=Unsigned  n_bits=fftsize + nochan - 1  bin_pt=0  load_pin=off  rst=on  en=off  explicit_period=on  period=1  dbl_ovrd=off  use_behavioral_HDL=off  use_rpm=off  implementation=Fabric  block_type=counter
  tvg2_chan : xps_library/software register  Tag=xps:sw_reg  SystemSampleTime=-1  io_dir=From Processor  arith_type=Unsigned  bitwidth=32  bin_pt=0  sample_period=1  gw_name=stg3_tvg2_tvg2_chan_user_data_out
      link override qdr_vacc_dram_buf_tv_tvg2_chan_user_data_out: arith_type=Unsigned  n_bits=32  bin_pt=0  period=1
      link override stg3_backup_tvg2_chan_user_data_out: arith_type=Unsigned  n_bits=32  bin_pt=0  period=1
      link override stg3_tvg2_chan_user_data_out: arith_type=Unsigned  n_bits=32  bin_pt=0  period=1
      link override stg3_tvg2_tvg2_chan_user_data_out: arith_type=Unsigned  n_bits=32  bin_pt=0  period=1
  sync_o : Outport
  Out1 : Outport  Port=2
  Out2 : Outport  Port=3
  wires:
  sync/1 -> progress/1, Delay4/1
  Delay3/1 -> sync_o/1
  Delay1/1 -> Out1/1
  progress/1 -> Slice1/1, Slice5/1, Slice6/1
  Slice1/1 -> Delay5/1, AddSub1/2
  Delay4/1 -> Delay3/1
  Constant3/1 -> AddSub1/1
  Delay2/1 -> Out2/1
  Convert1/1 -> Delay1/1
  Convert/1 -> Delay2/1
  tvg2_chan/1 -> Slice2/1, Slice3/1, Slice4/1
  Mux/1 -> Convert/1
  Constant1/1 -> Mux/3
  Logical1/1 -> Mux1/1
  Logical/1 -> Mux/1
  Delay5/1 -> Mux1/2
  Constant2/1 -> Mux1/3
  AddSub1/1 -> Mux/2
  Slice2/1 -> Logical/2, Inverter/1
  Inverter/1 -> Logical1/2
  Slice5/1 -> Relational/1
  Slice4/1 -> Relational/2
  Slice6/1 -> Relational1/1
  Slice3/1 -> Relational1/2
  Relational/1 -> Logical2/1
  Relational1/1 -> Logical2/2
  Logical2/1 -> Logical1/1, Logical/1
  Mux1/1 -> Convert1/1
  Constant/1 -> tvg2_chan/1

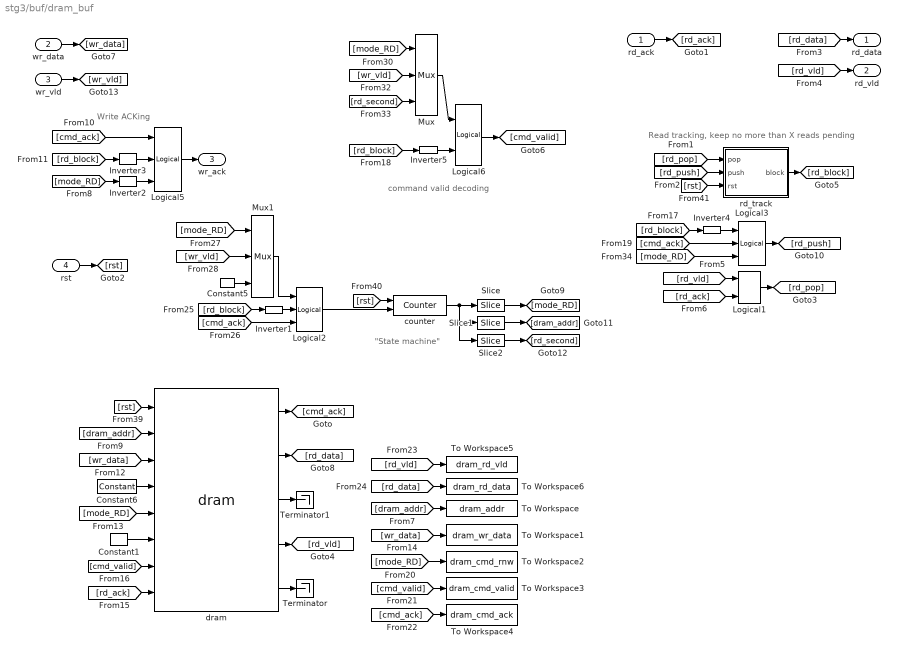
== system stg3/buf/dram_buf ==
  note: Write ACKing
  note: "State machine"
  note: command valid decoding
  note: Read tracking, keep no more than X reads pending
  rd_ack : Inport  OutDataType=sfix(16)  OutScaling=2^0
  wr_data : Inport  Port=2  OutDataType=sfix(16)  OutScaling=2^0
  wr_vld : Inport  Port=3  OutDataType=sfix(16)  OutScaling=2^0
  rst : Inport  Port=4  OutDataType=sfix(16)  OutScaling=2^0
  Constant1 : xbsIndex_r4/Constant  arith_type=Unsigned  const=0  n_bits=32  bin_pt=0  explicit_period=on  period=1  equ=P=C  opselect=C  inp2=PCIN>>17  opr=+  inp1=P  carry=CIN  dbl_ovrd=off  block_type=constant
  Constant5 : xbsIndex_r4/Constant  arith_type=Boolean  const=1  n_bits=32  bin_pt=0  explicit_period=on  period=1  equ=P=C  opselect=C  inp2=PCIN>>17  opr=+  inp1=P  carry=CIN  dbl_ovrd=off  block_type=constant
  Constant6 : xbsIndex_r4/Constant  arith_type=Unsigned  const=2^18 - 1  n_bits=18  bin_pt=0  explicit_period=on  period=1  equ=P=C  opselect=C  inp2=PCIN>>17  opr=+  inp1=P  carry=CIN  dbl_ovrd=off  block_type=constant
  Inverter{1..5} (5 alike) : xbsIndex_r4/Inverter  en=off  latency=0  dbl_ovrd=off  block_type=inv
  Logical1 : xbsIndex_r4/Logical  logical_function=AND  inputs=2  en=off  latency=0  precision=Full  arith_type=Unsigned  n_bits=16  bin_pt=0  align_bp=on  dbl_ovrd=off  block_type=logical
  Logical2 : xbsIndex_r4/Logical  logical_function=AND  inputs=3  en=off  latency=0  precision=Full  arith_type=Unsigned  n_bits=16  bin_pt=0  align_bp=on  dbl_ovrd=off  block_type=logical
  Logical3 : xbsIndex_r4/Logical  logical_function=AND  inputs=3  en=off  latency=0  precision=Full  arith_type=Unsigned  n_bits=16  bin_pt=0  align_bp=on  dbl_ovrd=off  block_type=logical
  Logical5 : xbsIndex_r4/Logical  logical_function=AND  inputs=3  en=off  latency=0  precision=Full  arith_type=Unsigned  n_bits=16  bin_pt=0  align_bp=on  dbl_ovrd=off  block_type=logical
  Logical6 : xbsIndex_r4/Logical  logical_function=AND  inputs=2  en=off  latency=0  precision=Full  arith_type=Unsigned  n_bits=16  bin_pt=0  align_bp=on  dbl_ovrd=off  block_type=logical
  Mux : xbsIndex_r4/Mux  inputs=2  en=off  latency=0  precision=Full  arith_type=Unsigned  n_bits=16  bin_pt=14  quantization=Truncate  overflow=Wrap  dbl_ovrd=off  block_type=mux
  Mux1 : xbsIndex_r4/Mux  inputs=2  en=off  latency=0  precision=Full  arith_type=Unsigned  n_bits=16  bin_pt=14  quantization=Truncate  overflow=Wrap  dbl_ovrd=off  block_type=mux
  Slice : xbsIndex_r4/Slice  nbits=1  boolean_output=on  mode=Upper Bit Location + Width  bit1=0  base1=MSB of Input  bit0=0  base0=LSB of Input  dbl_ovrd=off  block_type=slice
      settings: infoedit="Extracts a given range of bits from each input sample and presents it at the output.  The output type is ordinarily unsigned with binary point at zero, but can be Boolean when the slice is one bit wide.<P><P>Hardware notes: In hardware this block costs nothing."  block_version=10.1.3
  Slice1 : xbsIndex_r4/Slice  nbits=block_size - 1  boolean_output=off  mode=Lower Bit Location + Width  bit1=0  base1=LSB of Input  bit0=1  base0=LSB of Input  dbl_ovrd=off  block_type=slice
      settings: infoedit="Extracts a given range of bits from each input sample and presents it at the output.  The output type is ordinarily unsigned with binary point at zero, but can be Boolean when the slice is one bit wide.<P><P>Hardware notes: In hardware this block costs nothing."  block_version=10.1.3
  Slice2 : xbsIndex_r4/Slice  nbits=1  boolean_output=on  mode=Lower Bit Location + Width  bit1=0  base1=LSB of Input  bit0=0  base0=LSB of Input  dbl_ovrd=off  block_type=slice
      settings: infoedit="Extracts a given range of bits from each input sample and presents it at the output.  The output type is ordinarily unsigned with binary point at zero, but can be Boolean when the slice is one bit wide.<P><P>Hardware notes: In hardware this block costs nothing."  block_version=10.1.3
  Terminator : Terminator
  Terminator1 : Terminator
  To Workspace : ToWorkspace  VariableName=dram_addr  SampleTime=-1  SaveFormat=Array
  To Workspace1 : ToWorkspace  VariableName=dram_wr_data  SampleTime=-1  SaveFormat=Array
  To Workspace2 : ToWorkspace  VariableName=dram_cmd_rnw  SampleTime=-1  SaveFormat=Array
  To Workspace3 : ToWorkspace  VariableName=dram_cmd_valid  SampleTime=-1  SaveFormat=Array
  To Workspace4 : ToWorkspace  VariableName=dram_cmd_ack  SampleTime=-1  SaveFormat=Array
  To Workspace5 : ToWorkspace  VariableName=dram_rd_vld  SampleTime=-1  SaveFormat=Array
  To Workspace6 : ToWorkspace  VariableName=dram_rd_data  SampleTime=-1  SaveFormat=Array
  counter : xbsIndex_r4/Counter  cnt_type=Free Running  cnt_to=Inf  operation=Up  start_count=0  cnt_by_val=1  arith_type=Unsigned  n_bits=block_size+1  bin_pt=0  load_pin=off  rst=on  en=on  explicit_period=on  period=1  dbl_ovrd=off  use_behavioral_HDL=off  use_rpm=off  implementation=Fabric  block_type=counter
  dram : xps_library/dram  Tag=xps:dram  SystemSampleTime=-1  dimm=1  arith_type=Unsigned  bin_pt=0  ip_clock=266  sample_period=1  bram_fifos=off  disable_tag=off  use_sim=off  ram_depth=18  bank_mgt=off  wide_data=off  half_burst=off  use_sniffer=off
      link override convert_data_in: arith_type=Unsigned  n_bits=144  bin_pt=0
      link override convert_wr_be: n_bits=18
      link override dram_buffer_dram_block_buffer_dram_Mem_Rd_Dout: n_bits=144
      link override force_rd_dout: arith_type=Unsigned  bin_pt=0
      link override qdr_vacc_dram_buf_tv_buf_dram_buf_dram_Mem_Rd_Dout: n_bits=144
      link override qdr_vacc_dram_buf_tv_dram_block_buffer_dram_Mem_Rd_Dout: n_bits=144
      link override qdr_vacc_dram_buf_tv_tge_buffer_dram_block_buffer_dram_Mem_Rd_Dout: n_bits=144
      link override sim_wrapper/dram_sim: sim_method=Inactive  engine_block=ModelSim
      link override stg3_backup_buf_dram_buf_dram_Mem_Rd_Dout: n_bits=144
      link override stg3_buf_dram_buf_dram_Mem_Rd_Dout: n_bits=144
  rd_track : Subsystem  mask{max=16}
  rd_data : Outport  OutDataType=sfix(16)  OutScaling=2^0
  rd_vld : Outport  Port=2  OutDataType=sfix(16)  OutScaling=2^0
  wr_ack : Outport  Port=3  OutDataType=sfix(16)  OutScaling=2^0
  wires:
  [rd_data] -> To Workspace6/1
  [rd_vld] -> To Workspace5/1
  [cmd_ack] -> To Workspace4/1
  [cmd_valid] -> To Workspace3/1
  [mode_RD] -> To Workspace2/1
  [wr_data] -> To Workspace1/1
  [wr_data] -> dram/3
  wr_data/1 -> [wr_data]
  [dram_addr] -> To Workspace/1
  Logical6/1 -> [cmd_valid]
  Inverter5/1 -> Logical6/2
  [rd_block] -> Inverter5/1
  [cmd_valid] -> dram/7
  Constant1/1 -> dram/6
  [mode_RD] -> dram/5
  [rd_ack] -> dram/8
  Logical5/1 -> wr_ack/1
  [mode_RD] -> Inverter2/1
  Inverter3/1 -> Logical5/2
  [rd_block] -> Inverter3/1
  [cmd_ack] -> Logical5/1
  dram/4 -> [rd_vld]
  dram/2 -> [rd_data]
  dram/3 -> Terminator1/1
  dram/5 -> Terminator/1
  dram/1 -> [cmd_ack]
  [dram_addr] -> dram/2
  rd_ack/1 -> [rd_ack]
  rd_track/1(block) -> [rd_block]
  [rst] -> dram/1
  Constant6/1 -> dram/4
  [rd_pop] -> rd_track/1(pop)
  [rd_push] -> rd_track/2(push)
  [rd_data] -> rd_data/1
  [rd_vld] -> rd_vld/1
  [rd_vld] -> Logical1/1
  [rd_ack] -> Logical1/2
  Logical1/1 -> [rd_pop]
  counter/1 -> Slice/1, Slice1/1, Slice2/1
  Slice/1 -> [mode_RD]
  Slice1/1 -> [dram_addr]
  Inverter2/1 -> Logical5/3
  Slice2/1 -> [rd_second]
  Mux/1 -> Logical6/1
  [mode_RD] -> Mux/1
  wr_vld/1 -> [wr_vld]
  [wr_vld] -> Mux/2
  [rd_second] -> Mux/3
  [rd_block] -> Inverter4/1
  Inverter4/1 -> Logical3/1
  [cmd_ack] -> Logical3/2
  [mode_RD] -> Logical3/3
  Logical3/1 -> [rd_push]
  [rd_block] -> Inverter1/1
  Inverter1/1 -> Logical2/2
  [cmd_ack] -> Logical2/3
  Mux1/1 -> Logical2/1
  [mode_RD] -> Mux1/1
  [wr_vld] -> Mux1/2
  Constant5/1 -> Mux1/3
  Logical2/1 -> counter/2
  rst/1 -> [rst]
  [rst] -> rd_track/3(rst)
  [rst] -> counter/1
